simulink model "35-Bus_Network_Electricity_Transmission_Model"  (R2023b)
settings: Solver=VariableStepAuto  StartTime=0.0  StopTime=10  RelTol=1e-3
undefined symbols (not defined in the file): D1, D11, Delta
libraries: spsSeriesRLCBranchLib x47, spsLoadFlowBusLib x35, spsThreePhaseSeriesRLCLoadLib x27, spsDistributedParametersLineLib x22, spsGenericPowerSystemStabilizerLib x20, spsThreePhaseTransformerTwoWindingsLib x19, spsThreePhaseVIMeasurementLib x13, spsSynchronousMachinepuStandardLib x10, spsExcitationSystemLib x10, spsHydraulicTurbineandGovernorLib x10, spsThreePhaseParallelRLCLoadLib x4, spsGroundLib x3
(part 3 of 7)

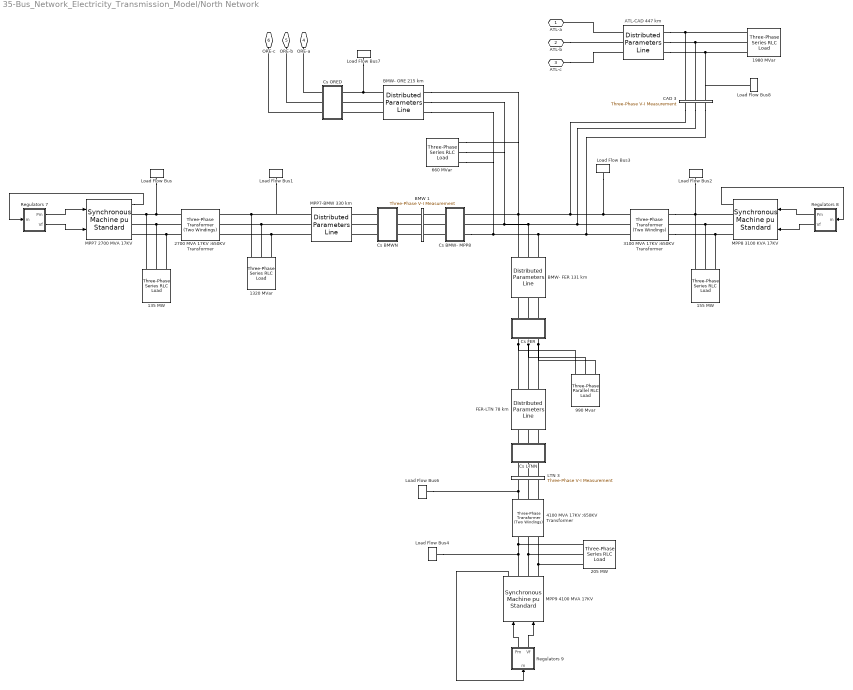
== system 35-Bus_Network_Electricity_Transmission_Model/North Network ==
  1320 MVar : spsThreePhaseSeriesRLCLoadLib/Three-Phase Series RLC Load  LConnTagsString=A|B|C  Configuration=Y (grounded)  NominalVoltage=1000  Vabc=[1e3 1e3 1e3]  Vabcp=[1e3 1e3 1e3]  NominalFrequency=60  UnbalancedPower=off  ActivePower=4400e3  InductivePower=1320e6  CapacitivePower=0  Pabc=[10e3 9e3 11e3]  QLabc=[100 90 110]  QCabc=[100 90 110]  Pabcp=[10e3 9e3 11e3]  QLabcp=[100 90 110]  QCabcp=[100 90 110]  Measurements=None  LoadType=constant Z
  135 MW : spsThreePhaseSeriesRLCLoadLib/Three-Phase Series RLC Load  LConnTagsString=A|B|C  Configuration=Y (grounded)  NominalVoltage=1000  Vabc=[1e3 1e3 1e3]  Vabcp=[1e3 1e3 1e3]  NominalFrequency=60  UnbalancedPower=off  ActivePower=135e6  InductivePower=0  CapacitivePower=0  Pabc=[10e3 9e3 11e3]  QLabc=[100 90 110]  QCabc=[100 90 110]  Pabcp=[10e3 9e3 11e3]  QLabcp=[100 90 110]  QCabcp=[100 90 110]  Measurements=None  LoadType=constant Z
  155 MW : spsThreePhaseSeriesRLCLoadLib/Three-Phase Series RLC Load  LConnTagsString=A|B|C  Configuration=Y (grounded)  NominalVoltage=1000  Vabc=[1e3 1e3 1e3]  Vabcp=[1e3 1e3 1e3]  NominalFrequency=60  UnbalancedPower=off  ActivePower=155e6  InductivePower=0  CapacitivePower=0  Pabc=[10e3 9e3 11e3]  QLabc=[100 90 110]  QCabc=[100 90 110]  Pabcp=[10e3 9e3 11e3]  QLabcp=[100 90 110]  QCabcp=[100 90 110]  Measurements=None  LoadType=constant Z
  1980 MVar : spsThreePhaseSeriesRLCLoadLib/Three-Phase Series RLC Load  LConnTagsString=A|B|C  Configuration=Y (grounded)  NominalVoltage=1000  Vabc=[1e3 1e3 1e3]  Vabcp=[1e3 1e3 1e3]  NominalFrequency=60  UnbalancedPower=off  ActivePower=6600e3  InductivePower=1980e6  CapacitivePower=0  Pabc=[10e3 9e3 11e3]  QLabc=[100 90 110]  QCabc=[100 90 110]  Pabcp=[10e3 9e3 11e3]  QLabcp=[100 90 110]  QCabcp=[100 90 110]  Measurements=None  LoadType=constant Z
  205 MW : spsThreePhaseSeriesRLCLoadLib/Three-Phase Series RLC Load  LConnTagsString=A|B|C  Configuration=Y (grounded)  NominalVoltage=1000  Vabc=[1e3 1e3 1e3]  Vabcp=[1e3 1e3 1e3]  NominalFrequency=60  UnbalancedPower=off  ActivePower=205e6  InductivePower=0  CapacitivePower=0  Pabc=[10e3 9e3 11e3]  QLabc=[100 90 110]  QCabc=[100 90 110]  Pabcp=[10e3 9e3 11e3]  QLabcp=[100 90 110]  QCabcp=[100 90 110]  Measurements=None  LoadType=constant Z
  "2700 MVA 17KV :650KV Transformer " : spsThreePhaseTransformerTwoWindingsLib/Three-Phase Transformer (Two Windings)  Winding1Connection=Yg  Winding2Connection=Delta (D1)  CoreType=Three single-phase transformers  SetSaturation=off  Hysteresis=off  DataFile='hysteresis'  SetInitialFlux=off  Measurements=None  UNITS=pu  NominalPower=[ 2700e6 , 60 ]  Winding1=[ 17e3 , 0.002 , 0.08 ]  Winding2=[ 6550e3 , 0.002 , 0.08 ]  Rm=500  Lm=500  L0=0.5  Saturation=[ 0,0 ; 0.0024,1.2 ; 1.0,1.52 ]  InitialFluxes=[ 0.8 , -0.8 , 0.7 ]  BreakLoop=off  DiscreteSolver=Trapezoidal iterative  DataType=off  TransfoNumber=1
  "3100 MVA 17KV :650KV Transformer " : spsThreePhaseTransformerTwoWindingsLib/Three-Phase Transformer (Two Windings)  Winding1Connection=Yg  Winding2Connection=Delta (D1)  CoreType=Three single-phase transformers  SetSaturation=off  Hysteresis=off  DataFile='hysteresis'  SetInitialFlux=off  Measurements=None  UNITS=pu  NominalPower=[ 3100e6 , 60 ]  Winding1=[ 17e3 , 0.002 , 0.08 ]  Winding2=[ 650e3 , 0.002 , 0.08 ]  Rm=500  Lm=500  L0=0.5  Saturation=[ 0,0 ; 0.0024,1.2 ; 1.0,1.52 ]  InitialFluxes=[ 0.8 , -0.8 , 0.7 ]  BreakLoop=off  DiscreteSolver=Trapezoidal iterative  DataType=off  TransfoNumber=1
  "4100 MVA 17KV :650KV Transformer " : spsThreePhaseTransformerTwoWindingsLib/Three-Phase Transformer (Two Windings)  Winding1Connection=Yg  Winding2Connection=Delta (D1)  CoreType=Three single-phase transformers  SetSaturation=off  Hysteresis=off  DataFile='hysteresis'  SetInitialFlux=off  Measurements=None  UNITS=pu  NominalPower=[ 4100e6 , 60 ]  Winding1=[ 17e3 , 0.002 , 0.08 ]  Winding2=[ 650e3 , 0.002 , 0.08 ]  Rm=500  Lm=500  L0=0.5  Saturation=[ 0,0 ; 0.0024,1.2 ; 1.0,1.52 ]  InitialFluxes=[ 0.8 , -0.8 , 0.7 ]  BreakLoop=off  DiscreteSolver=Trapezoidal iterative  DataType=off  TransfoNumber=1
  660 MVar : spsThreePhaseSeriesRLCLoadLib/Three-Phase Series RLC Load  LConnTagsString=A|B|C  Configuration=Y (grounded)  NominalVoltage=1000  Vabc=[1e3 1e3 1e3]  Vabcp=[1e3 1e3 1e3]  NominalFrequency=60  UnbalancedPower=off  ActivePower=2200e3  InductivePower=660e6  CapacitivePower=0  Pabc=[10e3 9e3 11e3]  QLabc=[100 90 110]  QCabc=[100 90 110]  Pabcp=[10e3 9e3 11e3]  QLabcp=[100 90 110]  QCabcp=[100 90 110]  Measurements=None  LoadType=constant Z
  990 Mvar : spsThreePhaseParallelRLCLoadLib/Three-Phase Parallel RLC Load  LConnTagsString=A|B|C  Configuration=Y (grounded)  NominalVoltage=1000  Vabc=[1e3 1e3 1e3]  Vabcp=[1e3 1e3 1e3]  NominalFrequency=60  UnbalancedPower=off  ActivePower=3300e3  InductivePower=990e6  CapacitivePower=0  Pabc=[10e3 9e3 11e3]  QLabc=[100 90 110]  QCabc=[100 90 110]  Pabcp=[10e3 9e3 11e3]  QLabcp=[100 90 110]  QCabcp=[100 90 110]  Measurements=None  LoadType=constant Z
  ATL-CAD 447 km : spsDistributedParametersLineLib/Distributed Parameters Line  Phases=3  Length=447  Frequency=60  Resistance=[0.01273 0.3864]/6  Inductance="[0.9337e-3  4.1264e-3]/6"  Capacitance=[12.74e-9 7.751e-9]*6  x1=[-0.00258 8.49668710026241e-13 -0.410901778452332 -0.465530911418911;-0.00252 9.63697655013433e-13 -0.398291866178216 -0.47447610558624;-0.00246 1.07723355447323e-12 -0.385478180425775 -0.48317854901064;-0.0024 1.19021832134158e-12 -0.372467276913411 -0.491633789361254;-0.00234 1.30259415052402e-12 -0.359265812259774 -0.499837500780882;-0.00228 1.41430354846988e-12 -0.345880540578116 -0.507785486099176;-0.00222 1.52528936258702e-12 -0.332318310020761 -0.515473678979984;-0.00216 1.63549481048215e-12 -0.318586059275462 -0.522898146001768;-0.0021 1.74486350901177e-12 -0.304690814015445 -0.53005508867001;-0.00204 1.85333950312881e-12 -0.290639683304939 -0.536940845360597;-0.00198 1.96086729451028e-12 -0.27643985596205 -0.543551893193172;-0.00192 2.0673918699512e-12 -0.262098596880829 -0.549884849833504;-0.00186 2.17285872951046e-12 -0.247623243314419 -0.555936475223958;-0.0018 2.27721391439388e-12 -0.233021201121178 -0.561703673241162;-0.00174 2.38040403456062e-12 -0.218299940975707 -0.567183493280046;-0.00168 2.48237629603847e-12 -0.203466994546713 -0.572373131763422;-0.00162 2.58307852793423e-12 -0.188529950643671 -0.577269933576348;-0.00156 2.6824592091253e-12 -0.173496451334247 -0.581871393424534;-0.0015 2.78046749461882e-12 -0.158374188034475 -0.586175157116098;-0.00144 2.87705324156497e-12 -0.143170897573686 -0.590179022766009;-0.00138 2.97216703491091e-12 -0.127894358236204 -0.593880941922619;-0.00132 3.06576021268245e-12 -0.112552385781832 -0.597279020615683;-0.00126 3.15778489088045e-12 -0.0971528294471658 -0.600371520325352;-0.0012 3.24819398797911e-12 -0.0817035679297762 -0.603156858871633;-0.00114 3.3369412490138e-12 -0.0662125053573254 -0.605633611223858;-0.00108 3.42398126924592e-12 -0.0506875672436673 -0.607800510229758;-0.00102 3.50926951739278e-12 -0.0351366964340088 -0.609656447263763;-0.00096 3.59276235841071e-12 -0.0195678490412032 -0.611200472794192;-0.0009 3.67441707581945e-12 -0.0039889903752558 -0.612431796869053;-0.00084 3.75419189355679e-12 0.0115919091318756 -0.613349789520197;-0.00078 3.83204599735189e-12 0.0271668780041013 -0.613953981085621;-0.00072 3.90793955560667e-12 0.0427279477995539 -0.614244062449757;-0.00066 3.98183373977439e-12 0.0582671571873906 -0.614219885201619;-0.0006 4.05369074422501e-12 0.073776556020957 -0.613881461710733;-0.00054 4.1234738055873e-12 0.089248209405229 -0.61322896512081;-0.00048 4.1911472215576e-12 0.104674201756452 -0.612262729261163;-0.00042 4.25667636916587e-12 0.120046640851899 -0.610983248475912;-0.00036 4.32002772248933e-12 0.13535766186768 -0.609391177371068;-0.0003 4.38116886980503e-12 0.150599431402528 -0.607487330479626;-0.00024 4.44006853017225e-12 0.165764151485512 -0.605272681844836;-0.00018 4.4966965694364e-12 0.180844063565627 -0.602748364521861;-0.00012 4.55102401564623e-12 0.195831452481207 -0.599915669998088;-6e-05 4.60302307387639e-12 0.210718650407149 -0.596776047532376]  x2=[-0.00258 1.36806566678117e-13 -0.210956808747724 -0.239084971192611;-0.00252 2.15529971640203e-13 -0.204464672732982 -0.243686885226569;-0.00246 2.94143107486261e-13 -0.197867928813597 -0.248164124547229;-0.0024 3.72605754283391e-13 -0.191169952005653 -0.252514398516225;-0.00234 4.50877769091666e-13 -0.184374169117848 -0.25673548145301;-0.00228 5.2891910650201e-13 -0.177484056998279 -0.260825213773558;-0.00222 6.06689839124167e-13 -0.170503140755621 -0.264781503095243;-0.00216 6.84150178014288e-13 -0.163434991955617 -0.268602325307345;-0.0021 7.61260493031696e-13 -0.156283226793798 -0.27228572560662;-0.00204 8.37981333114393e-13 -0.149051504245368 -0.275829819497412;-0.00198 9.14273446462953e-13 -0.141743524193211 -0.279232793755801;-0.00192 9.90097800622471e-13 -0.134363025534959 -0.282492907357275;-0.00186 1.06541560245229e-12 -0.126913784270099 -0.285608492367477;-0.0018 1.14018831797327e-12 -0.119399611568109 -0.288577954795545;-0.00174 1.21437769208252e-12 -0.11182435181859 -0.291399775409632;-0.00168 1.28794576812539e-12 -0.104191880664404 -0.294072510514171;-0.00162 1.36085490731477e-12 -0.0965061030188258 -0.296594792688496;-0.00156 1.43306780798787e-12 -0.0887709510677152 -0.29896533148644;-0.0015 1.50454752469036e-12 -0.0809903822577399 -0.301182914096551;-0.00144 1.57525748707837e-12 -0.0731683772716713 -0.303246405962589;-0.00138 1.64516151862858e-12 -0.0653089379917943 -0.305154751363989;-0.00132 1.71422385514677e-12 -0.0574160854524703 -0.306906973955978;-0.00126 1.78240916306545e-12 -0.0494938577829016 -0.308502177269103;-0.0012 1.84968255752117e-12 -0.0415463081411497 -0.309939545167873;-0.00114 1.91600962020226e-12 -0.0335775026404654 -0.31121834226831;-0.00108 1.98135641695787e-12 -0.0255915182689893 -0.312337914314189;-0.00102 2.0456895151593e-12 -0.0175924408038899 -0.313297688511763;-0.00096 2.10897600080479e-12 -0.00958436272100424 -0.31409717382282;-0.0009 2.17118349535886e-12 -0.0015713811010519 -0.3147359612159;-0.00084 2.23228017231786e-12 0.00644240446650752 -0.31521372387557;-0.00078 2.29223477349289e-12 0.0144528939809 -0.315530217369625;-0.00072 2.35101662500219e-12 0.0224559891276729 -0.315685279774147;-0.00066 2.40859565296433e-12 0.0304475953754693 -0.315678831756342;-0.0006 2.46494239888469e-12 0.0384236240708646 -0.315510876615137;-0.00054 2.52002803472689e-12 0.0463799945301984 -0.315181500279485;-0.00048 2.57382437766175e-12 0.0543126361273268 -0.314690871264405;-0.00042 2.62630390448619e-12 0.0622174903762302 -0.314039240584767;-0.00036 2.67743976570459e-12 0.0700905130074102 -0.313226941626869;-0.0003 2.72720579926545e-12 0.0779276760370118 -0.312254389977866;-0.00024 2.77557654394643e-12 0.085724969827615 -0.311122083213152;-0.00018 2.82252725238078e-12 0.093478405139639 -0.309830600641792;-0.00012 2.8680339037185e-12 0.101184015172311 -0.308380603010131;-6e-05 2.91207321591591e-12 0.108837857593156 -0.306772832163753]  x3=[-0.00258 -1.06703582362965e-15 -0.00161727071243747 -0.0149835486165627;-0.00252 -4.16919351273583e-16 -0.00123282394900618 -0.0150362004540804;-0.00246 2.33410424726374e-16 -0.000847746450062622 -0.0150811594936088;-0.0024 8.8362078364012e-16 -0.000462235228370651 -0.0151184027332724;-0.00234 1.53337906583352e-15 -7.64875185947201e-05 -0.0151479111187418;-0.00228 2.18235284296325e-15 0.000309299323609049 -0.0151696695529815;-0.00222 2.83021008805327e-15 0.000694927922563665 -0.0151836669039748;-0.00216 3.47661934536598e-15 0.0010802009835523 -0.015189896010418;-0.0021 4.12124989998106e-15 0.00146492139375794 -0.0151883536853853;-0.00204 4.76377194699537e-15 0.0018488923231099 -0.0151790407179586;-0.00198 5.4038567602572e-15 0.00223191732498575 -0.0151619618728242;-0.00192 6.0411768605487e-15 0.00261380043671704 -0.0151371258878348;-0.00186 6.67540618313023e-15 0.00299434627984744 -0.0151045454695393;-0.0018 7.30622024456114e-15 0.0033733601600919 -0.0150642372866817;-0.00174 7.93329630871152e-15 0.00375064816694594 -0.0150162219616731;-0.00168 8.55631355187989e-15 0.00412601727289375 -0.014960524060041;-0.00162 9.17495322693262e-15 0.00449927543216472 -0.0148971720778611;-0.00156 9.78889882638081e-15 0.00487023167898754 -0.0148261984271781;-0.0015 1.03978362443114e-14 0.00523869622529186 -0.0147476394194231;-0.00144 1.10014539370894e-14 0.00560448055780734 -0.014661535246836;-0.00138 1.15994430827498e-14 0.00596739753451055 -0.0145679299619027;-0.00132 1.21914977389959e-14 0.00632726148037028 -0.0144668714548164;-0.00126 1.27773149997258e-14 0.0066838882823423 -0.0143584114289769;-0.0012 1.33565951500042e-14 0.00703709548356502 -0.0142426053745373;-0.00114 1.39290418194023e-14 0.00738670237670778 -0.014119512540015;-0.00108 1.44943621336266e-14 0.00773253009642405 -0.0139891959019786;-0.00102 1.50522668643583e-14 0.00807440171086225 -0.0138517221328282;-0.00096 1.56024705772282e-14 0.00841214231218739 -0.0137071615666843;-0.0009 1.61446917778503e-14 0.0087455791060671 -0.0135555881634035;-0.00084 1.66786530558393e-14 0.00907454150007642 -0.01339707947074;-0.00078 1.72040812267388e-14 0.00939886119097605 -0.0132317165846696;-0.00072 1.77207074717879e-14 0.00971837225081939 -0.0130595841079005;-0.00066 1.82282674754534e-14 0.0100329112118443 -0.0128807701065884;-0.0006 1.87265015606587e-14 0.0103423171501064 -0.0126953660652805;-0.00054 1.92151548216397e-14 0.0106464317678105 -0.0125034668401103;-0.00048 1.96939772543587e-14 0.0109450994742987 -0.0123051706102671;-0.00042 2.01627238844115e-14 0.0112381674656536 -0.0121005788277663;-0.00036 2.06211548923607e-14 0.0115254858028757 -0.0118897961655443;-0.0003 2.10690357364319e-14 0.0118069074885945 -0.0116729304639057;-0.00024 2.15061372725093e-14 0.0120822885422756 -0.0114500926753509;-0.00018 2.19322358713704e-14 0.0123514880738835 -0.01122139680781;-0.00012 2.23471135330985e-14 0.0126143683559635 -0.0109869598663146;-6e-05 2.27505579986159e-14 0.0128707948941058 -0.010746901793136]  x4=[-0.00258 -2.43849292593164e-14 -0.0174366757595381 0.00359918610184665;-0.00252 -2.3635764122212e-14 -0.0174954192556241 0.00325087591105733;-0.00246 -2.2874506491444e-14 -0.0175452117719408 0.00290090251208264;-0.0024 -2.21015458404827e-14 -0.0175860278337167 0.00254944495778025;-0.00234 -2.13172776302797e-14 -0.0176178465587004 0.00219668306032913;-0.00228 -2.05221031069432e-14 -0.0176406516678443 0.00184279729923431;-0.00222 -1.97164290964522e-14 -0.0176544314936332 0.00148796872899022;-0.00216 -1.89006677965178e-14 -0.0176591789860536 0.00113237888644989;-0.0021 -1.80752365656945e-14 -0.0176548917162006 0.000776209697947285;-0.00204 -1.72405577098522e-14 -0.0176415718775207 0.000419643386220505;-0.00198 -1.63970582661167e-14 -0.0176192262846895 6.2862377183218e-05;-0.00192 -1.55451697843894e-14 -0.0175878663701251 -0.000293950793407798;-0.00186 -1.46853281065587e-14 -0.0175475081781394 -0.000650613573341321;-0.0018 -1.38179731435151e-14 -0.0174981723567291 -0.00100694348734877;-0.00174 -1.29435486500844e-14 -0.0174398841470121 -0.00136275823046191;-0.00168 -1.20625019979951e-14 -0.0173726733703134 -0.00171787576128347;-0.00162 -1.11752839469942e-14 -0.0172965744129084 -0.00207211439512286;-0.00156 -1.02823484142305e-14 -0.0172116262084298 -0.00242529289694944;-0.0015 -9.38415224202209e-15 -0.0171178722179486 -0.00277723057411567;-0.00144 -8.4811549641275e-15 -0.0170153604077389 -0.00312774736880287;-0.00138 -7.57381857063954e-15 -0.0169041432247368 -0.00347666395014207;-0.00132 -6.66260727162276e-15 -0.0167842775697084 -0.003823801805963;-0.00126 -5.747987259615e-15 -0.0166558247681374 -0.00416898333412428;-0.0012 -4.83042647111462e-15 -0.0165188505388509 -0.00451203193337786;-0.00114 -3.9103943471756e-15 -0.0163734249603953 -0.00485277209372155;-0.00108 -2.98836159323279e-15 -0.016219622435184 -0.00519102948619319;-0.00102 -2.0647999382803e-15 -0.0160575216514306 -0.00552663105206049;-0.00096 -1.14018189352628e-15 -0.0158872055428915 -0.00585940509136115;-0.0009 -2.14980510647385e-16 -0.0157087612464348 -0.00618918135074772;-0.00084 7.10330860233135e-16 -0.01552228005746 -0.00651579111059233;-0.00078 1.63527881272016e-15 -0.0153278573831889 -0.00683906727130677;-0.00072 2.55939012635011e-15 -0.0151255926938544 -0.00715884443883379;-0.00066 3.48219200869933e-15 -0.0149155894718089 -0.00747495900926565;-0.0006 4.4032123372734e-15 -0.0146979551585812 -0.00778724925254702;-0.00054 5.3219799010537e-15 -0.0144728010999074 -0.00809555539521897;-0.00048 6.23802464157774e-15 -0.0142402424887643 -0.00839971970216205;-0.00042 7.15087789342971e-15 -0.0140003983064345 -0.00869958655729653;-0.00036 8.06007262401837e-15 -0.0137533912616335 -0.00899500254319843;-0.0003 8.96514367251957e-15 -0.0134993477277296 -0.00928581651959069;-0.00024 9.86562798786109e-15 -0.0132383976780889 -0.00957187970066936;-0.00018 1.07610648656282e-14 -0.0129706746195787 -0.00985304573122517;-0.00012 1.16509961837684e-14 -0.0126963155242626 -0.0101291707615215;-6e-05 1.25349666369753e-14 -0.0124154607593233 -0.0104001135208907]  x5=0.00252797080447097  V1=[6.404e-19 2.341e-08 2.341e-08;377 377 377;-1.588 0.8733 -0.6975]  V2=[3.447e-16 8.016e-05 8.016e-05;377 377 377;2.581 0.8892 -0.6816]  I1=[4.995e-19 5.332e-07 5.332e-07;377 377 377;1.203 -0.6479 -2.219]  I2=[4.022e-19 5.225e-07 5.225e-07;377 377 377;-2.95 1.909 0.3385]  nHarmo=1  Measurements=None  Decoupling=off  VsMag0=0  VrMag0=0  VsAngle0=0  VrAngle0=0  IsMag0=0  IrMag0=0  IsAngle0=0  IrAngle0=0
      settings: LibrarySourceBlock=sps_lib/Power Grid Elements/Distributed Parameters Line
  BMW 1 : spsThreePhaseVIMeasurementLib/Three-Phase V-I Measurement  VoltageMeasurement=no  SetLabelV=off  LabelV=Vabc  Vpu=off  VpuLL=off  CurrentMeasurement=no  SetLabelI=off  LabelI=Iabc  Ipu=off  Pbase=100e6  Vbase=500e3  OutputType=Complex  PhasorSimulation=off  PSBequivalent=0
  BMW- FER 131 km : spsDistributedParametersLineLib/Distributed Parameters Line  Phases=3  Length=131  Frequency=60  Resistance=[0.01273 0.3864]/6  Inductance="[0.9337e-3  4.1264e-3]/6"  Capacitance=[12.74e-9 7.751e-9]*6  x1=[-0.00078 3.83204599735189e-12 0.0271668780041014 -0.613953981085621;-0.00072 3.90793955560667e-12 0.042727947799554 -0.614244062449757;-0.00066 3.98183373977439e-12 0.0582671571873907 -0.614219885201619;-0.0006 4.05369074422501e-12 0.073776556020957 -0.613881461710733;-0.00054 4.1234738055873e-12 0.089248209405229 -0.61322896512081;-0.00048 4.1911472215576e-12 0.104674201756452 -0.612262729261163;-0.00042 4.25667636916587e-12 0.120046640851899 -0.610983248475912;-0.00036 4.32002772248933e-12 0.13535766186768 -0.609391177371068;-0.0003 4.38116886980503e-12 0.150599431402528 -0.607487330479626;-0.00024 4.44006853017225e-12 0.165764151485512 -0.605272681844836;-0.00018 4.4966965694364e-12 0.180844063565627 -0.602748364521861;-0.00012 4.55102401564623e-12 0.195831452481207 -0.599915669998088;-6e-05 4.60302307387639e-12 0.210718650407149 -0.596776047532376]  x2=[-0.00078 -7.09060014169606e-13 -0.219701275891047 1.44554590759906;-0.00072 -7.13899186668542e-13 -0.256406755704317 1.44323531985658;-0.00066 -7.18373115152239e-13 -0.292981053083518 1.44018634625654;-0.0006 -7.22479510676215e-13 -0.329405455942293 1.43640054671018;-0.00054 -7.26216272332642e-13 -0.365661328883096 1.43187985810248;-0.00048 -7.29581488325211e-13 -0.401730122731397 1.42662659330129;-0.00042 -7.32573436947236e-13 -0.43759338402579 1.42064343997393;-0.00036 -7.35190587462518e-13 -0.473232764459119 1.41393345921221;-0.0003 -7.37431600888494e-13 -0.508630030265815 1.40650008396626;-0.00024 -7.39295330681287e-13 -0.543767071550624 1.39834711728823;-0.00018 -7.40780823322296e-13 -0.578625911553968 1.38947873038651;-0.00012 -7.41887318806037e-13 -0.613188715849183 1.37989946049171;-6e-05 -7.42614251028976e-13 -0.647437801466945 1.36961420853531]  x3=[-0.00078 9.4310978366865e-14 0.299338778582478 0.00472729268801372;-0.00072 9.16500661766956e-14 0.298635072053784 0.0107468954083704;-0.00066 8.89422641191717e-14 0.297778578304086 0.0167609998184564;-0.0006 8.61889575558604e-14 0.296769735531413 0.0227665289913276;-0.00054 8.33915551292747e-14 0.295609059878367 0.0287604103872897;-0.00048 8.0551488042186e-14 0.29429714516806 0.0347395774258665;-0.00042 7.76702093253946e-14 0.292834662600299 0.0407009710547185;-0.00036 7.47491930943319e-14 0.291222360408189 0.0466415413147115;-0.0003 7.17899337948759e-14 0.289461063475324 0.0525582489003313;-0.00024 6.87939454387649e-14 0.287551672913759 0.0584480667146489;-0.00018 6.57627608290015e-14 0.285495165602988 0.0643079814180392;-0.00012 6.26979307756419e-14 0.28329259369015 0.0701349949698612;-6e-05 5.96010233023729e-14 0.280945084051735 0.0759261261623108]  x4=[-0.00078 -7.35205011779578e-14 -0.301818709052308 0.0138174520161851;-0.00072 -7.02251680599393e-14 -0.301590131627545 0.00777590378326555;-0.00066 -6.68939064483295e-14 -0.301207255118696 0.00173037725428826;-0.0006 -6.35284206781235e-14 -0.300670275412458 -0.00431603456766602;-0.00054 -6.01304325940282e-14 -0.299979467237571 -0.0103602382265843;-0.00048 -5.67016806695352e-14 -0.299135184024262 -0.0163991413961907;-0.00042 -5.32439191174851e-14 -0.298137857723423 -0.0224296544620376;-0.00036 -4.975891699258e-14 -0.296987998585619 -0.0284486921022092;-0.0003 -4.62484572863024e-14 -0.295686194900032 -0.03445317486583;-0.00024 -4.27143360147039e-14 -0.294233112693481 -0.040440030748568;-0.00018 -3.91583612995301e-14 -0.292629495389673 -0.0464061967643291;-0.00012 -3.55823524431521e-14 -0.290876163428852 -0.0523486205123377;-6e-05 -3.1988138997778e-14 -0.288974013848048 -0.0582642617388009]  x5=0.000740859452764423  V1=[1.271e-18 2.341e-08 2.341e-08;377 377 377;2.226 1.284 -0.2866]  V2=[3.351e-20 3.07e-09 3.07e-09;377 377 377;-0.6702 -1.817 2.896]  I1=[5.66e-21 5.705e-10 5.705e-10;377 377 377;-2.518 2.745 1.174]  I2=[6.071e-21 5.74e-10 5.74e-10;377 377 377;0.8934 -0.2657 -1.836]  nHarmo=1  Measurements=None  Decoupling=off  VsMag0=0  VrMag0=0  VsAngle0=0  VrAngle0=0  IsMag0=0  IrMag0=0  IsAngle0=0  IrAngle0=0
      settings: LibrarySourceBlock=sps_lib/Power Grid Elements/Distributed Parameters Line
  BMW- ORE 215 km : spsDistributedParametersLineLib/Distributed Parameters Line  Phases=3  Length=215  Frequency=60  Resistance=[0.01273 0.3864]/6  Inductance="[0.9337e-3  4.1264e-3]/6"  Capacitance=[12.74e-9 7.751e-9]*6  x1=[-0.00126 3.15778489088045e-12 -0.0971528294471658 -0.600371520325352;-0.0012 3.24819398797911e-12 -0.0817035679297762 -0.603156858871633;-0.00114 3.3369412490138e-12 -0.0662125053573254 -0.605633611223858;-0.00108 3.42398126924592e-12 -0.0506875672436673 -0.607800510229758;-0.00102 3.50926951739278e-12 -0.0351366964340088 -0.609656447263763;-0.00096 3.59276235841071e-12 -0.0195678490412032 -0.611200472794192;-0.0009 3.67441707581945e-12 -0.0039889903752558 -0.612431796869053;-0.00084 3.75419189355679e-12 0.0115919091318756 -0.613349789520197;-0.00078 3.83204599735189e-12 0.0271668780041013 -0.613953981085621;-0.00072 3.90793955560667e-12 0.0427279477995539 -0.614244062449757;-0.00066 3.98183373977439e-12 0.0582671571873907 -0.614219885201619;-0.0006 4.05369074422501e-12 0.073776556020957 -0.613881461710733;-0.00054 4.1234738055873e-12 0.089248209405229 -0.61322896512081;-0.00048 4.1911472215576e-12 0.104674201756452 -0.612262729261163;-0.00042 4.25667636916587e-12 0.120046640851899 -0.610983248475912;-0.00036 4.32002772248933e-12 0.13535766186768 -0.609391177371068;-0.0003 4.38116886980503e-12 0.150599431402528 -0.607487330479626;-0.00024 4.44006853017225e-12 0.165764151485512 -0.605272681844836;-0.00018 4.4966965694364e-12 0.180844063565627 -0.602748364521861;-0.00012 4.55102401564623e-12 0.195831452481207 -0.599915669998088;-6e-05 4.60302307387639e-12 0.210718650407149 -0.596776047532376]  x2=[-0.00126 9.80688247419646e-13 -0.0217497081183819 -0.116994984678567;-0.0012 9.70196253744707e-13 -0.01873459817215 -0.117583207929365;-0.00114 9.59207889739186e-13 -0.0157099032593175 -0.118111273438298;-0.00108 9.47728777253151e-13 -0.012677170869692 -0.118578911037295;-0.00102 9.35764789212659e-13 -0.00963795260520237 -0.118985881474319;-0.00096 9.2332204661506e-13 -0.00659380338607103 -0.119331976535774;-0.0009 9.10406915397384e-13 -0.00354628065528788 -0.119617019153032;-0.00084 8.97026003179404e-13 -0.000496943581793759 -0.119840863493024;-0.00078 8.83186155883063e-13 0.00255264773721926 -0.120003395032847;-0.00072 8.68894454229969e-13 0.00560093307448242 -0.120104530618364;-0.00066 8.54158210118767e-13 0.00864635287089134 -0.12014421850674;-0.0006 8.38984962884239e-13 0.0116873490334053 -0.120122438392918;-0.00054 8.2338247544004e-13 0.0147223657321963 -0.120039201420007;-0.00048 8.07358730307047e-13 0.0177498501966408 -0.11989455017358;-0.00042 7.90921925529354e-13 0.0207682535097451 -0.119688558659888;-0.00036 7.74080470480005e-13 0.0237760314006006 -0.119421332267995;-0.0003 7.56842981558595e-13 0.026771645034461 -0.119093007715861;-0.00024 7.39218277782969e-13 0.0297535618000387 -0.118703752980394;-0.00018 7.21215376277246e-13 0.0327202560936168 -0.118253767211509;-0.00012 7.02843487658492e-13 0.0356702100995767 -0.11774328063024;-6e-05 6.84112011324397e-13 0.0386019145669399 -0.117172554410955]  x3=[-0.00126 8.23335356372037e-14 0.0397730894754066 -0.0196193340624535;-0.0012 8.19147265452958e-14 0.0401962258486255 -0.0188418777567085;-0.00114 8.14540083656774e-14 0.0405987970899594 -0.0180547815981452;-0.00108 8.0951616810282e-14 0.0409805972365225 -0.0172584482797023;-0.00102 8.04078089119125e-14 0.041341430952305 -0.0164532852202201;-0.00096 7.98228628927383e-14 0.0416811136281105 -0.0156397043559974;-0.0009 7.91970780219512e-14 0.0419994714760055 -0.0148181219300378;-0.00084 7.85307744626543e-14 0.0422963416182323 -0.0139889582790912;-0.00078 7.78242931080605e-14 0.0425715721705407 -0.0131526376186029;-0.00072 7.7077995407085e-14 0.0428250223198944 -0.0123095878256761;-0.00066 7.62922631794216e-14 0.0430565623965139 -0.0114602402201627;-0.0006 7.54674984201967e-14 0.0432660739402175 -0.0106050293439917;-0.00054 7.4604123094301e-14 0.0434534497610282 -0.00974439273884993;-0.00048 7.37025789205045e-14 0.0436185939940137 -0.00887877072232729;-0.00042 7.27633271454652e-14 0.0437614221483329 -0.00800860616264228;-0.00036 7.17868483077466e-14 0.0438818611504629 -0.00713434425206245;-0.0003 7.07736419919654e-14 0.0439798493815847 -0.00625643227913573;-0.00024 6.97242265731945e-14 0.0440553367091088 -0.00537531939984943;-0.00018 6.86391389517532e-14 0.0441082845123235 -0.00449145640783368;-0.00012 6.75189342785187e-14 0.0441386657021542 -0.00360529550372711;-6e-05 6.63641856709008e-14 0.044146464735023 -0.00271729006382264]  x4=[-0.00126 -5.76168660268718e-14 -0.0449169150785053 0.00432896818364091;-0.0012 -5.64242514949969e-14 -0.0449416289200406 0.00342684884060788;-0.00114 -5.52027692734569e-14 -0.0449433497937946 0.00252297625838711;-0.00108 -5.39530442951266e-14 -0.0449220768193364 0.00161781287489331;-0.00102 -5.26757159423974e-14 -0.044877820880313 0.000711821788438974;-0.00096 -5.13714377200567e-14 -0.0448106046188804 -0.000194533479195285;-0.0009 -5.00408769209434e-14 -0.04472046242412 -0.00110078921990702;-0.00084 -4.86847142845482e-14 -0.0446074404144443 -0.00200648177651361;-0.00078 -4.7303643648735e-14 -0.0444715964140018 -0.00291114777996781;-0.00072 -4.58983715947602e-14 -0.0443129999230933 -0.00381432438642596;-0.00066 -4.44696170857732e-14 -0.0441317320826141 -0.0047155495140474;-0.0006 -4.3018111098981e-14 -0.0439278856325407 -0.00561436207940411;-0.00054 -4.15445962516674e-14 -0.0437015648644837 -0.00651030223337952;-0.00048 -4.00498264212554e-14 -0.04345288556833 -0.00740291159643578;-0.00042 -3.85345663596107e-14 -0.0431819749730026 -0.00829173349312922;-0.00036 -3.69995913017795e-14 -0.0428889716813677 -0.00917631318575396;-0.0003 -3.54456865693644e-14 -0.0425740255993237 -0.0100561981069941;-0.00024 -3.38736471687395e-14 -0.0422372978591054 -0.0109309380914655;-0.00018 -3.228427738431e-14 -0.0418789607368469 -0.0118000856060288;-0.00012 -3.06783903670258e-14 -0.0414991975644413 -0.0126631959787556;-6e-05 -2.90568077183584e-14 -0.0410982026357446 -0.0135198276264307]  x5=0.00121591436904085  V1=[1.271e-18 2.341e-08 2.341e-08;377 377 377;2.047 1.175 -0.3959]  V2=[2.813e-15 0.004697 0.004697;377 377 377;-0.9882 1.143 -0.4279]  I1=[7.991e-18 6.252e-05 6.252e-05;377 377 377;-2.327 -0.3924 -1.963]  I2=[7.132e-18 6.19e-05 6.19e-05;377 377 377;0.3426 2.469 0.8982]  nHarmo=1  Measurements=None  Decoupling=off  VsMag0=0  VrMag0=0  VsAngle0=0  VrAngle0=0  IsMag0=0  IrMag0=0  IsAngle0=0  IrAngle0=0
      settings: LibrarySourceBlock=sps_lib/Power Grid Elements/Distributed Parameters Line
  CAD 3 : spsThreePhaseVIMeasurementLib/Three-Phase V-I Measurement  VoltageMeasurement=no  SetLabelV=off  LabelV=Vabc  Vpu=off  VpuLL=off  CurrentMeasurement=no  SetLabelI=off  LabelI=Iabc  Ipu=off  Pbase=100e6  Vbase=500e3  OutputType=Complex  PhasorSimulation=off  PSBequivalent=0
  Cs BMW- MPP8 : Subsystem
  Cs BMWN : Subsystem
  Cs FER : Subsystem
  Cs LTNN : Subsystem
  Cs ORED : Subsystem
  FER-LTN 78 km : spsDistributedParametersLineLib/Distributed Parameters Line  Phases=3  Length=78  Frequency=60  Resistance=[0.01273 0.3864]/6  Inductance="[0.9337e-3  4.1264e-3]/6"  Capacitance=[12.74e-9 7.751e-9]*6  x1=[-0.00048 1.87803979252904e-15 0 0;-0.00042 1.88389486263069e-15 0 0;-0.00036 1.88878609731025e-15 0 0;-0.0003 1.89271099412166e-15 0.00120896465466599 0.0289970143907712;-0.00024 1.89566754501521e-15 0.000361453270260355 0.029119674620409;-0.00018 1.89765423736482e-15 -0.000486243040317235 0.0292274366864414;-0.00012 1.89867005474197e-15 -0.00133369057997066 0.0293202454558039;-6e-05 1.89871447743573e-15 -0.0021804557788796 0.0293980534458155]  x2=[-0.00048 -6.86836632330327e-13 0 0;-0.00042 -6.90156589214769e-13 0 0;-0.00036 -6.9312344923554e-13 0 0;-0.0003 -6.95735694492235e-13 10.6282553538029 131.520825361648;-0.00024 -6.97991988511909e-13 6.76701955965324 132.166977147993;-0.00018 -6.99891176932852e-13 2.90232163325667 132.745509866663;-0.00012 -7.01432288095173e-13 -0.963861174516213 133.256127529631;-6e-05 -7.02614533537927e-13 -4.8295508531021 133.698568895465]  x3=[-0.00048 -6.65778771132694e-15 0 0;-0.00042 -7.36378375328101e-15 0 0;-0.00036 -8.06601234739983e-15 0 0;-0.0003 -8.76411422055894e-15 37.3040582475667 -5.52153422510258;-0.00024 -9.45773221094061e-15 37.3165687614738 -4.86576636571784;-0.00018 -1.01465114507644e-14 37.3099874292716 -4.20750909035138;-0.00012 -1.08300995478439e-14 37.2843176180913 -3.54709917558847;-6e-05 -1.15081467658776e-14 37.2395724610827 -2.88487449934447]  x4=[-0.00048 -4.03991572477091e-15 0 0;-0.00042 -3.37545062423122e-15 0 0;-0.00036 -2.70925858078102e-15 0 0;-0.0003 -2.04168043057954e-15 -36.8775374239324 8.39533043253787;-0.00024 -1.37305771894386e-15 -36.9751878040426 7.75719596326579;-0.00018 -7.03732525607983e-16 -37.0539209948494 7.11509276920239;-0.00012 -3.40472897085214e-17 -37.1136967149974 6.46934936220648;-6e-05 6.35655365413476e-16 -37.1544843821238 5.82029611653703]  x5=0.000441122422256679  V1=[6.391e-24 5.815e-13 5.815e-13;377 377 377;2.579 1.39 -0.1804]  V2=[2.845e-25 1.398e-13 1.398e-13;377 377 377;-0.3188 -1.706 3.006]  I1=[5.031e-26 2.613e-14 2.613e-14;377 377 377;-2.041 2.924 1.353]  I2=[5.244e-26 2.622e-14 2.622e-14;377 377 377;1.254 -0.1553 -1.726]  nHarmo=1  Measurements=None  Decoupling=off  VsMag0=0  VrMag0=0  VsAngle0=0  VrAngle0=0  IsMag0=0  IrMag0=0  IsAngle0=0  IrAngle0=0
      settings: LibrarySourceBlock=sps_lib/Power Grid Elements/Distributed Parameters Line
  LTN 3 : spsThreePhaseVIMeasurementLib/Three-Phase V-I Measurement  VoltageMeasurement=no  SetLabelV=off  LabelV=Vabc  Vpu=off  VpuLL=off  CurrentMeasurement=no  SetLabelI=off  LabelI=Iabc  Ipu=off  Pbase=100e6  Vbase=500e3  OutputType=Complex  PhasorSimulation=off  PSBequivalent=0
  Load Flow Bus : spsLoadFlowBusLib/Load Flow Bus  LConnTagsString=a  Phases=single  Connectors=on one side  ID=BUS_13  Vbase=17e3  Vref=1  Vangle=0  VLF=1  VLFb=1  VLFc=1  angleLF=0  angleLFb=0  angleLFc=0
  Load Flow Bus1 : spsLoadFlowBusLib/Load Flow Bus  LConnTagsString=a  Phases=single  Connectors=on one side  ID=BUS_14  Vbase=650e3  Vref=1  Vangle=0  VLF=1  VLFb=1  VLFc=1  angleLF=0  angleLFb=0  angleLFc=0
  Load Flow Bus2 : spsLoadFlowBusLib/Load Flow Bus  LConnTagsString=a  Phases=single  Connectors=on one side  ID=BUS_15  Vbase=17e3  Vref=1  Vangle=0  VLF=1  VLFb=1  VLFc=1  angleLF=0  angleLFb=0  angleLFc=0
  Load Flow Bus3 : spsLoadFlowBusLib/Load Flow Bus  LConnTagsString=a  Phases=single  Connectors=on one side  ID=BUS_16  Vbase=650e3  Vref=1  Vangle=0  VLF=1  VLFb=1  VLFc=1  angleLF=0  angleLFb=0  angleLFc=0
  Load Flow Bus4 : spsLoadFlowBusLib/Load Flow Bus  LConnTagsString=a  Phases=single  Connectors=on one side  ID=BUS_17  Vbase=17e3  Vref=1  Vangle=0  VLF=1  VLFb=1  VLFc=1  angleLF=0  angleLFb=0  angleLFc=0
  Load Flow Bus6 : spsLoadFlowBusLib/Load Flow Bus  LConnTagsString=a  Phases=single  Connectors=on one side  ID=BUS_18  Vbase=650e3  Vref=1  Vangle=0  VLF=1  VLFb=1  VLFc=1  angleLF=0  angleLFb=0  angleLFc=0
  Load Flow Bus7 : spsLoadFlowBusLib/Load Flow Bus  LConnTagsString=a  Phases=single  Connectors=on one side  ID=BUS_19  Vbase=650e3  Vref=1  Vangle=0  VLF=1  VLFb=1  VLFc=1  angleLF=0  angleLFb=0  angleLFc=0
  Load Flow Bus8 : spsLoadFlowBusLib/Load Flow Bus  LConnTagsString=a  Phases=single  Connectors=on one side  ID=BUS_20  Vbase=650e3  Vref=1  Vangle=0  VLF=1  VLFb=1  VLFc=1  angleLF=0  angleLFb=0  angleLFc=0
  MPP7 2700 MVA 17KV : spsSynchronousMachinepuStandardLib/Synchronous Machine pu Standard  PresetModel=No  MechanicalLoad=Mechanical power Pm  ShowDetailedParameters=on  RotorType=Salient-pole  Units=per unit standard parameters  MeasurementBus=off  NominalParameters=[2700e6 17000 60]  Reactances1=[ 1.81, 0.3, 0.23, 1.76, 0.65, 0.25, 0.15 ]  Reactances2=[2.24 0.17 0.12 1.02 0.13 0.08]  dAxisTimeConstants=Short-circuit  qAxisTimeConstants=Open-circuit  TimeConstants1="[ 4.4849  0.0681  0.1  ]"  TimeConstants2=[ 8.0, 0.03, 1.0, 0.07 ]  TimeConstants3="[  4.49  0.0681  0.0513  ]"  TimeConstants4=[ 8.0, 0.03, 0.3371, 0.0295 ]  TimeConstants5=[ 1.01, 0.053, 0.1 ]  TimeConstants6=[ 1.3201, 0.023, 1.0, 0.07 ]  TimeConstants7=[0.012 0.003 0.003]  TimeConstants8=[ 1.3201, 0.0231, 0.3371, 0.0295 ]  StatorResistance=0.037875  Mechanical=[3.8 0 28]  PolePairs=20  InitialConditions=[ 0 -78.876 0.604539 0.604539 0.604539 -42.1129 -162.113 77.8871 1.28555]  SetSaturation=off  Saturation=[0.6404,0.7127,0.8441,0.9214,0.9956,1.082,1.19,1.316,1.457;0.7,0.7698,0.8872,0.9466,0.9969,1.046,1.1,1.151,1.201]  LoadFlowParameters=[1,0,0,0,0]  TsPowergui=0  TsBlock=-1  IterativeModel=Trapezoidal non iterative  IterativeDiscreteModel=Trapezoidal non iterative  BusType=PV  Pref=2200e6  Qref=0  Qmin=-inf  Qmax=inf  PLF=0  QLF=0
  MPP7-BMW 330 km : spsDistributedParametersLineLib/Distributed Parameters Line  Phases=3  Length=330  Frequency=60  Resistance=[0.01273 0.3864]/6  Inductance="[0.9337e-3  4.1264e-3]/6"  Capacitance=[12.74e-9 7.751e-9]*6  x1=[-0.00192 -2.54461091903707e-11 0 0;-0.00186 -2.551290054946e-11 0 0;-0.0018 -2.5566639037204e-11 0 0;-0.00174 -2.56072971599993e-11 0 0;-0.00168 -2.56348541163992e-11 0 0;-0.00162 -2.56492958077555e-11 0 0;-0.00156 -2.5650614845432e-11 0 0;-0.0015 -2.56388105545848e-11 0 0;-0.00144 -2.56138889745071e-11 0 0;-0.00138 -2.55758628555397e-11 0 0;-0.00132 -2.55247516525479e-11 0 0;-0.00126 -2.54605815149674e-11 0 0;-0.0012 -2.53833852734265e-11 0 0;-0.00114 -2.52932024229486e-11 -0.0758769501998661 -1.15148332725884;-0.00108 -2.51900791027465e-11 -0.0468436520514124 -1.15437647985176;-0.00102 -2.50740680726163e-11 -0.0177863878249981 -1.15667903210716;-0.00096 -2.49452286859446e-11 0.0112799762460821 -1.15838980599677;-0.0009 -2.48036268593423e-11 0.040340569272885 -1.15950792625705;-0.00084 -2.46493350389205e-11 0.0693805233190397 -1.16003282083701;-0.00078 -2.44824321632255e-11 0.0983849810074598 -1.15996422119089;-0.00072 -2.43030036228524e-11 0.127339103121651 -1.15930216241553;-0.00066 -2.41111412167579e-11 0.156228076197729 -1.15804698323244;-0.0006 -2.39069431052944e-11 0.185037120103262 -1.15619932581448;-0.00054 -2.36905137599886e-11 0.213751495599056 -1.15376013545733;-0.00048 -2.34619639100928e-11 0.242356511880029 -1.15073066009584;-0.00042 -2.32214104859334e-11 0.27083753409129 -1.14711244966559;-0.00036 -2.29689765590871e-11 0.299179990815609 -1.14290735530989;-0.0003 -2.27047912794153e-11 0.327369381528415 -1.13811752843271;-0.00024 -2.24289898089886e-11 0.355391284016541 -1.13274541959799;-0.00018 -2.21417132529355e-11 0.383231361756887 -1.12679377727587;-0.00012 -2.18431085872504e-11 0.410875371251258 -1.12026564643655;-6e-05 -2.15333285835979e-11 0.438309169313593 -1.11316436699238]  x2=[-0.00192 -4.3780775583102e-14 0 0;-0.00186 -5.24132754308771e-14 0 0;-0.0018 -6.10189596784557e-14 0 0;-0.00174 -6.95934254987621e-14 0 0;-0.00168 -7.81322860366447e-14 0 0;-0.00162 -8.66311726532723e-14 0 0;-0.00156 -9.50857371612105e-14 0 0;-0.0015 -1.03491654049035e-13 0 0;-0.00144 -1.11844622694341e-13 0 0;-0.00138 -1.20140369564026e-13 0 0;-0.00132 -1.28374650400704e-13 0 0;-0.00126 -1.36543252394146e-13 0 0;-0.0012 -1.44641996336633e-13 0 0;-0.00114 -1.52666738761118e-13 -0.0113185196194015 -0.089265721629606;-0.00108 -1.60613374061096e-13 -0.00868174098497981 -0.0897784329469309;-0.00102 -1.68477836591111e-13 -0.00604052061145007 -0.0902452119590454;-0.00096 -1.76256102746812e-13 -0.00339620979595952 -0.0906658198531819;-0.0009 -1.8394419302351e-13 -0.000750161416782615 -0.0910400414385698;-0.00084 -1.9153817405216e-13 0.00189627075883651 -0.0913676852565311;-0.00078 -1.99034160611746e-13 0.00454173276729635 -0.0916485836784346;-0.00072 -2.06428317617034e-13 0.00718487114135087 -0.091882592991457;-0.00066 -2.13716862080673e-13 0.00982433360256832 -0.0920695934721098;-0.0006 -2.20896065048638e-13 0.0124587697531819 -0.0922094894474919;-0.00054 -2.27962253508034e-13 0.0150868317669781 -0.0923022093442372;-0.00048 -2.34911812266277e-13 0.0177071750788698 -0.0923477057251332;-0.00042 -2.41741185800693e-13 0.0203184590728001 -0.0923459553133908;-0.00036 -2.48446880077591e-13 0.0229193477676269 -0.0922969590045531;-0.0003 -2.5502546433987e-13 0.0255085105006348 -0.0922007418660369;-0.00024 -2.61473572862264e-13 0.0280846226083276 -0.0920573531243082;-0.00018 -2.67787906673306e-13 0.0306463661041497 -0.0918668661396968;-0.00012 -2.73965235243141e-13 0.0331924303527933 -0.0916293783688638;-6e-05 -2.80002398136332e-13 0.0357215127407428 -0.0913450113149411]  x3=[-0.00192 -1.43265957905022e-13 0 0;-0.00186 -1.38844681705055e-13 0 0;-0.0018 -1.34352370000373e-13 0 0;-0.00174 -1.29791321140652e-13 0 0;-0.00168 -1.25163868642769e-13 0 0;-0.00162 -1.20472379996925e-13 0 0;-0.00156 -1.15719255455401e-13 0 0;-0.0015 -1.1090692680454e-13 0 0;-0.00144 -1.06037856120601e-13 0 0;-0.00138 -1.01114534510117e-13 0 0;-0.00132 -9.61394808353958e-14 0 0;-0.00126 -9.11152404258258e-14 0 0;-0.0012 -8.60443837756379e-14 0 0;-0.00114 -8.09295052287929e-14 0.0538872721716838 -0.0287868216848857;-0.00108 -7.57732216516676e-14 0.054529426045907 -0.0277008176877285;-0.00102 -7.05781710942171e-14 0.0551436816581772 -0.0266006414403899;-0.00096 -6.53470114403002e-14 0.0557297247439729 -0.0254868558133671;-0.0009 -6.00824190478564e-14 0.0562872554728228 -0.0243600306399673;-0.00084 -5.47870873796323e-14 0.0568159886017038 -0.0232207424247704;-0.00078 -4.94637256251559e-14 0.0573156536209774 -0.022069574048679;-0.00072 -4.4115057314665e-14 0.057785994892787 -0.0209071144707055;-0.00066 -3.87438189256995e-14 0.0582267717818471 -0.0197339584266497;-0.0006 -3.3352758483068e-14 0.0586377587785565 -0.0185507061248212;-0.00054 -2.79446341529085e-14 0.0590187456143736 -0.0173579629389616;-0.00048 -2.2522212831559e-14 0.0593695373693934 -0.0161563390985241;-0.00042 -1.70882687299621e-14 0.0596899545720721 -0.0149464493764691;-0.00036 -1.16455819543281e-14 0.0599798332910482 -0.0137289127747343;-0.0003 -6.19693708378066e-15 0.0602390252190126 -0.0125043522075429;-0.00024 -7.45121745714919e-16 0.0604673977485858 -0.0112733941827083;-0.00018 4.7070748104042e-15 0.0606648340401618 -0.0100366684811014;-0.00012 1.01568631400736e-14 0.0608312330816856 -0.00879480783444329;-6e-05 1.56014550308832e-14 0.0609665097403329 -0.0075484476015877]  x4=[-0.00192 -2.96013848554736e-14 0 0;-0.00186 -3.61605871346774e-14 0 0;-0.0018 -4.27012889893322e-14 0 0;-0.00174 -4.92201440755111e-14 0 0;-0.00168 -5.57138172264972e-14 0 0;-0.00162 -6.21789861591173e-14 0 0;-0.00156 -6.86123431734828e-14 0 0;-0.0015 -7.50105968452703e-14 0 0;-0.00144 -8.13704737096754e-14 0 0;-0.00138 -8.76887199361772e-14 0 0;-0.00132 -9.39621029932583e-14 0 0;-0.00126 -1.00187413302228e-13 0 0;-0.0012 -1.06361465879302e-13 0 0;-0.00114 -1.12481101965098e-13 -0.0625021075044613 0.00239969122183952;-0.00108 -1.18543190640717e-13 -0.0624583311056341 0.00110441566605453;-0.00102 -1.24544630429578e-13 -0.0623825998705161 -0.000191424929192462;-0.00096 -1.3048235088419e-13 -0.0622749525446064 -0.00148716758790855;-0.0009 -1.36353314157054e-13 -0.062135444202266 -0.00278214938420698;-0.00084 -1.42154516554876e-13 -0.0619641462185408 -0.00407570778147223;-0.00078 -1.47882990075314e-13 -0.0617611462326444 -0.00536718097132606;-0.00072 -1.53535803925467e-13 -0.0615265481031206 -0.00665590821222085;-0.00066 -1.59110066021316e-13 -0.0612604718547074 -0.00794123016748723;-0.0006 -1.64602924467372e-13 -0.0609630536169299 -0.00922248924266287;-0.00054 -1.70011569015759e-13 -0.0606344455544542 -0.01049902992193;-0.00048 -1.75333232503984e-13 -0.0602748157892372 -0.0117701991034892;-0.00042 -1.80565192270675e-13 -0.0598843483145119 -0.0130353464336988;-0.00036 -1.85704771548539e-13 -0.0594632429006533 -0.0142938246398075;-0.0003 -1.90749340833849e-13 -0.0590117149929724 -0.0155449898611109;-0.00024 -1.95696319231746e-13 -0.0585299956014899 -0.016788201978363;-0.00018 -2.00543175776672e-13 -0.0580183311827478 -0.0180228249412726;-0.00012 -2.05287430727259e-13 -0.057476983513717 -0.0192482270939188;-6e-05 -2.0992665683501e-13 -0.0569062295578681 -0.0204637814979174]  x5=0.00186628717108595  V1=[7.602e-19 2.561e-08 2.561e-08;377 377 377;2.359 1.029 -0.5418]  V2=[1.596e-23 1.649e-13 1.649e-13;377 377 377;-0.06951 1.06 -0.5113]  I1=[1.208e-21 2.221e-10 2.221e-10;377 377 377;-2.873 2.204 0.633]  I2=[1.433e-21 2.255e-10 2.255e-10;377 377 377;1.006 -0.507 -2.078]  nHarmo=1  Measurements=None  Decoupling=off  VsMag0=0  VrMag0=0  VsAngle0=0  VrAngle0=0  IsMag0=0  IrMag0=0  IsAngle0=0  IrAngle0=0
      settings: LibrarySourceBlock=sps_lib/Power Grid Elements/Distributed Parameters Line
  MPP8 3100 KVA 17KV : spsSynchronousMachinepuStandardLib/Synchronous Machine pu Standard  PresetModel=No  MechanicalLoad=Mechanical power Pm  ShowDetailedParameters=on  RotorType=Salient-pole  Units=per unit standard parameters  MeasurementBus=off  NominalParameters=[3100e6 17000 60]  Reactances1=[ 1.81, 0.3, 0.23, 1.76, 0.65, 0.25, 0.15 ]  Reactances2=[2.24 0.17 0.12 1.02 0.13 0.08]  dAxisTimeConstants=Short-circuit  qAxisTimeConstants=Open-circuit  TimeConstants1="[ 4.4849  0.0681  0.1  ]"  TimeConstants2=[ 8.0, 0.03, 1.0, 0.07 ]  TimeConstants3="[  4.49  0.0681  0.0513  ]"  TimeConstants4=[ 8.0, 0.03, 0.3371, 0.0295 ]  TimeConstants5=[ 1.01, 0.053, 0.1 ]  TimeConstants6=[ 1.3201, 0.023, 1.0, 0.07 ]  TimeConstants7=[0.012 0.003 0.003]  TimeConstants8=[ 1.3201, 0.0231, 0.3371, 0.0295 ]  StatorResistance=0.037875  Mechanical=[3.8 0 28]  PolePairs=20  InitialConditions="[  0 -93.496 0.604539 0.604539 0.604539 -42.1129 -162.113 77.8871 1.28555]"  SetSaturation=off  Saturation=[0.6404,0.7127,0.8441,0.9214,0.9956,1.082,1.19,1.316,1.457;0.7,0.7698,0.8872,0.9466,0.9969,1.046,1.1,1.151,1.201]  LoadFlowParameters=[1,0,0,0,0]  TsPowergui=0  TsBlock=-1  IterativeModel=Trapezoidal non iterative  IterativeDiscreteModel=Trapezoidal non iterative  BusType=PV  Pref=2400e6  Qref=0  Qmin=-inf  Qmax=inf  PLF=0  QLF=0
  MPP9 4100 MVA 17KV : spsSynchronousMachinepuStandardLib/Synchronous Machine pu Standard  PresetModel=No  MechanicalLoad=Mechanical power Pm  ShowDetailedParameters=on  RotorType=Salient-pole  Units=per unit standard parameters  MeasurementBus=off  NominalParameters="[4100e6  17000   60]"  Reactances1=[ 1.81, 0.3, 0.23, 1.76, 0.65, 0.25, 0.15 ]  Reactances2=[2.24 0.17 0.12 1.02 0.13 0.08]  dAxisTimeConstants=Short-circuit  qAxisTimeConstants=Open-circuit  TimeConstants1="[ 4.4849  0.0681  0.1  ]"  TimeConstants2=[ 8.0, 0.03, 1.0, 0.07 ]  TimeConstants3="[  4.49  0.0681  0.0513  ]"  TimeConstants4=[ 8.0, 0.03, 0.3371, 0.0295 ]  TimeConstants5=[ 1.01, 0.053, 0.1 ]  TimeConstants6=[ 1.3201, 0.023, 1.0, 0.07 ]  TimeConstants7=[0.012 0.003 0.003]  TimeConstants8=[ 1.3201, 0.0231, 0.3371, 0.0295 ]  StatorResistance=0.037875  Mechanical=[3.8 0 28]  PolePairs=20  InitialConditions=[ 0 -85.876 0.604539 0.604539 0.604539 -42.1129 -162.113 77.8871 1.28555]  SetSaturation=off  Saturation=[0.6404,0.7127,0.8441,0.9214,0.9956,1.082,1.19,1.316,1.457;0.7,0.7698,0.8872,0.9466,0.9969,1.046,1.1,1.151,1.201]  LoadFlowParameters=[1,0,0,0,0]  TsPowergui=0  TsBlock=-1  IterativeModel=Trapezoidal non iterative  IterativeDiscreteModel=Trapezoidal non iterative  BusType=PV  Pref=3500e6  Qref=0  Qmin=-inf  Qmax=inf  PLF=0  QLF=0
  Regulators 7 : Subsystem
  Regulators 8 : Subsystem
  Regulators 9 : Subsystem
  ATL-a : PMIOPort  Side=Right
  ATL-b : PMIOPort  Port=2  Side=Right
  ATL-c : PMIOPort  Port=3  Side=Right
  ORE-a : PMIOPort  Port=4  Side=Left
  ORE-b : PMIOPort  Port=5  Side=Left
  ORE-c : PMIOPort  Port=6  Side=Left
  wires:
  Regulators 8/2(Vf) -> MPP8 3100 KVA 17KV/2
  MPP8 3100 KVA 17KV/1 -> Regulators 8/1(m)
  Regulators 8/1(Pm) -> MPP8 3100 KVA 17KV/1
  Regulators 7/1(Pm) -> MPP7 2700 MVA 17KV/1
  Regulators 7/2(Vf) -> MPP7 2700 MVA 17KV/2
  Regulators 9/1(Pm) -> MPP9 4100 MVA 17KV/1
  Regulators 9/2(Vf) -> MPP9 4100 MVA 17KV/2
  MPP9 4100 MVA 17KV/1 -> Regulators 9/1(m)
  MPP7 2700 MVA 17KV/1 -> Regulators 7/1(m)
  connections:
  ATL-c/RConn1 -- ATL-CAD 447 km/RConn3
  1320 MVar/LConn2 -- MPP7-BMW 330 km/RConn2 -- "2700 MVA 17KV :650KV Transformer "/LConn2
  1320 MVar/LConn1 -- MPP7-BMW 330 km/RConn1 -- Load Flow Bus1/LConn1 -- "2700 MVA 17KV :650KV Transformer "/LConn1
  Cs FER/RConn3 -- FER-LTN 78 km/LConn3 -- 990 Mvar/LConn3
  MPP8 3100 KVA 17KV/RConn2 -- "3100 MVA 17KV :650KV Transformer "/RConn2 -- 155 MW/LConn2
  1320 MVar/LConn3 -- MPP7-BMW 330 km/RConn3 -- "2700 MVA 17KV :650KV Transformer "/LConn3
  Cs FER/LConn3 -- BMW- FER 131 km/RConn3
  "3100 MVA 17KV :650KV Transformer "/RConn3 -- 155 MW/LConn3 -- MPP8 3100 KVA 17KV/RConn3
  Cs FER/RConn2 -- FER-LTN 78 km/LConn2 -- 990 Mvar/LConn2
  ATL-CAD 447 km/RConn1 -- ATL-a/RConn1
  "3100 MVA 17KV :650KV Transformer "/RConn1 -- MPP8 3100 KVA 17KV/RConn1 -- Load Flow Bus2/LConn1 -- 155 MW/LConn1
  Cs FER/RConn1 -- FER-LTN 78 km/LConn1 -- 990 Mvar/LConn1
  Cs FER/LConn2 -- BMW- FER 131 km/RConn2
  Cs FER/LConn1 -- BMW- FER 131 km/RConn1
  ATL-b/RConn1 -- ATL-CAD 447 km/RConn2
  "2700 MVA 17KV :650KV Transformer "/RConn1 -- 135 MW/LConn1 -- MPP7 2700 MVA 17KV/RConn1 -- Load Flow Bus/LConn1
  "2700 MVA 17KV :650KV Transformer "/RConn2 -- 135 MW/LConn2 -- MPP7 2700 MVA 17KV/RConn2
  "2700 MVA 17KV :650KV Transformer "/RConn3 -- 135 MW/LConn3 -- MPP7 2700 MVA 17KV/RConn3
  "4100 MVA 17KV :650KV Transformer "/LConn1 -- LTN 3/RConn1 -- Load Flow Bus6/LConn1
  "4100 MVA 17KV :650KV Transformer "/LConn2 -- LTN 3/RConn2
  "4100 MVA 17KV :650KV Transformer "/LConn3 -- LTN 3/RConn3
  MPP9 4100 MVA 17KV/RConn1 -- Load Flow Bus4/LConn1 -- 205 MW/LConn1 -- "4100 MVA 17KV :650KV Transformer "/RConn1
  MPP9 4100 MVA 17KV/RConn2 -- 205 MW/LConn2 -- "4100 MVA 17KV :650KV Transformer "/RConn2
  MPP9 4100 MVA 17KV/RConn3 -- 205 MW/LConn3 -- "4100 MVA 17KV :650KV Transformer "/RConn3
  BMW- FER 131 km/LConn1 -- BMW- ORE 215 km/LConn1 -- 660 MVar/LConn1 -- CAD 3/RConn1 -- Load Flow Bus3/LConn1 -- "3100 MVA 17KV :650KV Transformer "/LConn1 -- Cs BMW- MPP8/LConn1
  "3100 MVA 17KV :650KV Transformer "/LConn2 -- BMW- ORE 215 km/LConn2 -- 660 MVar/LConn2 -- Cs BMW- MPP8/LConn2 -- BMW- FER 131 km/LConn2 -- CAD 3/RConn2
  BMW- FER 131 km/LConn3 -- 660 MVar/LConn3 -- BMW- ORE 215 km/LConn3 -- Cs BMW- MPP8/LConn3 -- CAD 3/RConn3 -- "3100 MVA 17KV :650KV Transformer "/LConn3
  Cs BMWN/RConn1 -- MPP7-BMW 330 km/LConn1
  Cs BMWN/RConn2 -- MPP7-BMW 330 km/LConn2
  Cs BMWN/RConn3 -- MPP7-BMW 330 km/LConn3
  BMW 1/RConn1 -- Cs BMWN/LConn1
  BMW 1/RConn2 -- Cs BMWN/LConn2
  BMW 1/RConn3 -- Cs BMWN/LConn3
  Cs BMW- MPP8/RConn1 -- BMW 1/LConn1
  Cs BMW- MPP8/RConn2 -- BMW 1/LConn2
  Cs BMW- MPP8/RConn3 -- BMW 1/LConn3
  ATL-CAD 447 km/LConn1 -- 1980 MVar/LConn1 -- CAD 3/LConn1
  ATL-CAD 447 km/LConn2 -- 1980 MVar/LConn2 -- CAD 3/LConn2
  ATL-CAD 447 km/LConn3 -- Load Flow Bus8/LConn1 -- CAD 3/LConn3 -- 1980 MVar/LConn3
  Cs ORED/RConn1 -- ORE-a/RConn1
  Cs ORED/RConn2 -- ORE-b/RConn1
  Cs ORED/RConn3 -- ORE-c/RConn1
  BMW- ORE 215 km/RConn1 -- Load Flow Bus7/LConn1 -- Cs ORED/LConn1
  BMW- ORE 215 km/RConn2 -- Cs ORED/LConn2
  BMW- ORE 215 km/RConn3 -- Cs ORED/LConn3
  Cs LTNN/RConn1 -- FER-LTN 78 km/RConn1
  Cs LTNN/RConn2 -- FER-LTN 78 km/RConn2
  Cs LTNN/RConn3 -- FER-LTN 78 km/RConn3
  LTN 3/LConn1 -- Cs LTNN/LConn1
  LTN 3/LConn2 -- Cs LTNN/LConn2
  LTN 3/LConn3 -- Cs LTNN/LConn3
